simulink model "single_thruster_sol"  (R2022b)
settings: Solver=VariableStepAuto  StartTime=0.0  StopTime=31  RelTol=1e-3
libraries: simulink x1, MarineRoboticsLib x1, MarineRoboticsLibEx x1
settings Model: Creator=dnad  LastModifiedBy=dnad

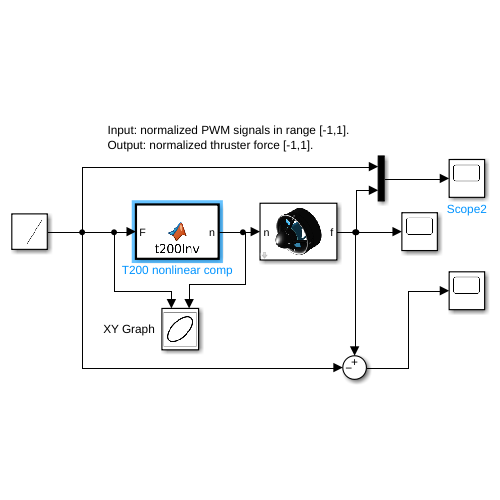
[thumbnail: Simulink's stored preview of the top-level diagram]
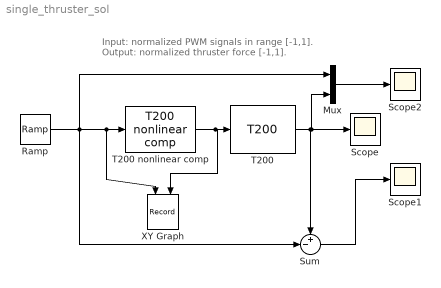
== system single_thruster_sol ==
  note: Input: normalized PWM signals in range [-1,1].
      | Output: normalized thruster force [-1,1].
  Mux : Mux  Inputs=2
  Ramp : simulink/Sources/Ramp  slope=0.1  start=0  InitialOutput=-1.5
  Scope : Scope
  Scope1 : Scope
  Scope2 : Scope
  Sum : Sum  Inputs=+-|
  T200 : MarineRoboticsLib/T200  Keff=1  Tm=0
  T200 nonlinear comp : MarineRoboticsLibEx/T200 nonlinear comp  SystemSampleTime=-1  VariantActivationTime=update diagram  Latency=0  AutoFrameSizeCalculation=off
      settings: LibrarySourceBlock=|
      | simulink/User-Defined
      | Functions/MATLAB Function
  XY Graph : Record  FileSettingsInternal="{\"entries\":[{\"content\":{\"excelSettings\":{\"content\":{},\"type\":\"Streamout.ExcelSettings\"}},\"type\":\"Streamout.FileSettingStorage\",\"uuid\":\"ff5869e4-6c58-4188-b555-8163ff53dcd8\"}],\"packageUris\":[\"http://schema.mathworks.com/mf0/streamout_blocks/R2020a\"],\"version\":\"1.0\"}"  Layout=[1 1]  SignalsInternal="{\"entries\":[{\"content\":{\"signals\":[{\"content\":{\"blockPath\":[\"single_thruster_sol/XY Graph\"],\"channel\":[],\"dimensions\":[1],\"domain\":\"single_thruster_sol/XY Graph\",\"lineColor\":\"#a2142f\",\"plots\":[1],\"port\":1,\"sid\":[\"\"],\"signalID\":19,\"signalName\":\"Ramp\"},\"type\":\"RecordBlkView.Signal\",\"uuid\":\"8c470111-8aac-4115-96b8-0f334b7c2fc6\"},{\"content\":{\"blockPath\":[\"single_thruster_sol/XY Graph\"],\"channel\":[],\"dimensions\":[1],\"domain\":\"single_thruster_sol/XY Graph\",\"lineColor\":\"#139fff\",\"plots\":[1],\"port\":2,\"sid\":[\"\"],\"signalID\":23,\"signalName\":\"T200 nonlinear comp\"},\"type\":\"RecordBlkView.Signal\",\"uuid\":\"42c76fbe-66c3-4034-b031-2b6e34b76f8f\"}]},\"type\":\"RecordBlkView.InputSignals\",\"uuid\":\"3c92e4f2-72a5-4e98-8e0c-8b7606768c79\"}],\"packageUris\":[\"http://schema.mathworks.com/mf0/streamout_blocks/R2020a\"],\"version\":\"1.0\"}"  VisualizationBindings="{\"xyplotplugin\":{\"info\":[{\"series\":[{\"bindingParametersList\":[{\"parameter\":\"X-Axis\",\"signalID\":19,\"signalName\":\"Ramp\"},{\"parameter\":\"Y-Axis\",\"signalID\":23,\"signalName\":\"T200 nonlinear comp\"}],\"seriesID\":4241}],\"subplotID\":1}]}}"  CompatibilityTag=XY
  wires:
  Ramp/1 -> T200 nonlinear comp/1, XY Graph/1, Sum/2, Mux/1
  Mux/1 -> Scope2/1
  Sum/1 -> Scope1/1
  T200 nonlinear comp/1 -> XY Graph/2, T200/1
  T200/1 -> Mux/2, Scope/1, Sum/1
